simulink model "Sliding_mode_observer"  (R2024b)
settings: Solver=VariableStepAuto  StartTime=0.0  StopTime=10  FixedStep=1e-5  RelTol=1e-3  EnableMultiTasking=on
values from neighbouring files (symbols this model uses):
  Ad = Ts / Ld    (= 0.0178571428571)    [init_params.m]
  Aq = Ts / Lq    (= 0.0178571428571)    [init_params.m]
  Bd = 1-(Rs*Ts/Ld)    (= 0.908928571429)    [init_params.m]
  Bq = 1-(Rs*Ts/Lq)    (= 0.908928571429)    [init_params.m]
  Bs = 1E-5    (= 1e-05)    [init_params.m]
  J = 0.0002    [init_params.m]
  k_sat = 1    [init_params.m]
  k_smo = 8    [init_params.m]
  Ki_current = Rs * bw_current    (= 6408.84901332)    [init_params.m]
  Kp_current = Ld * bw_current    (= 3.51858377202)    [init_params.m]
  Ld = 2.8e-3    (= 0.0028)    [init_params.m]
  Lq = 2.8e-3    (= 0.0028)    [init_params.m]
  Pn = 7    [init_params.m]
  psi_f = 0.0078    [init_params.m]
  Rs = 5.1    [init_params.m]
  Ts = 50e-6    (= 5e-05)    [init_params.m]
undefined symbols (not defined in the file or in its folder): DiscIntNeverNeededParam
libraries: slpidlib x4, eeGeneralControl x4, spsPWMGenerator2LevelLib x1, spsDCVoltageSourceLib x1, spsGroundLib x1, spsPermanentMagnetSynchronousMachineLib x1, spsThreePhaseVIMeasurementLib x1, spsTwoLevelConverterLib x1, spspowerguiLib x1
settings Model: Creator=yangchaojie  LastModifiedBy=yangchaojie
settings SolverCC: PositivePriorityOrder=on  AutoInsertRateTranBlk=on
settings OptimizationCC: DefaultParameterBehavior=Inlined  UseDivisionForNetSlopeComputation=on  GainParamInheritBuiltInType=on  UseFloatMulNetSlope=on  InlineInvariantSignals=on  PassReuseOutputArgsAs=Individual arguments  ZeroExternalMemoryAtStartup=off  ZeroInternalMemoryAtStartup=off  NoFixptDivByZeroProtection=on  EfficientFloat2IntCast=on  LifeSpan=1  MaxStackSize=512  OptimizeBlockOrder=speed  DifferentSizesBufferReuse=on  EfficientTunableParamExpr=on
settings DebuggingCC: ParameterTunabilityLossMsg=error
settings HardwareCC: ProdBitPerPointer=32  ProdBitPerSizeT=32  ProdBitPerPtrDiffT=32  ProdLargestAtomicInteger=Long  ProdLargestAtomicFloat=Double  ProdWordSize=32  ProdLongLongMode=on  ProdHWDeviceType=ARM Compatible->ARM Cortex-M
settings SFSimCC: MATLABDynamicMemAlloc=off
settings RTWCC: Description=Embedded Coder  SystemTargetFile=ert.tlc  GenCodeOnly=on  TemplateMakefile=ert_default_tmf  GenerateReport=on  Toolchain=GNU Tools for ARM Embedded Processors  LaunchReport=on
settings CodeAppCC: ForceParamTrailComments=on  IgnoreCustomStorageClasses=off  OperatorAnnotations=on  SimulinkDataObjDesc=on  SFDataObjDesc=on  CustomSymbolStrGlobalVar=rt$N$M  CustomSymbolStrType=$N$M  CustomSymbolStrFcn=$N$M$F  CustomSymbolStrMacro=$N$M  InsertBlockDesc=on
settings ERTTargetCC: TargetLangStandard=C99 (ISO)  CodeReplacementLibrary=ARM Cortex-M  IncludeMdlTerminateFcn=off  CombineSignalStateStructs=on  SupportAbsoluteTime=off  SupportComplex=off  SupportNonInlinedSFcns=on  ExtModeTransport=3  ExtModeStaticAlloc=on  ExtModeStaticAllocSize=2048  ExtModeMexFile=ext_xcp  ExtModeIntrfLevel=Level2 - Open  ERTCustomFileTemplate=example_file_process.tlc  ERTFilePackagingFormat=CompactWithDataFile

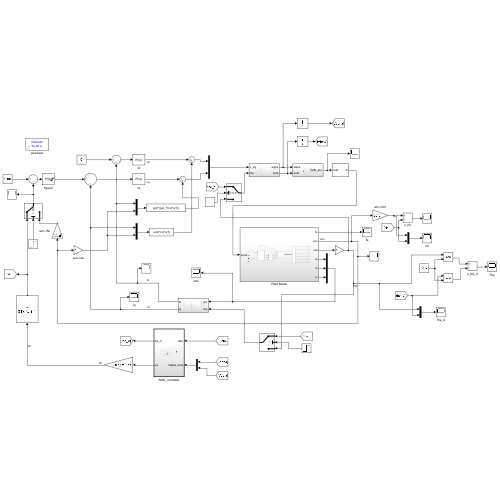
[thumbnail: Simulink's stored preview of the top-level diagram]
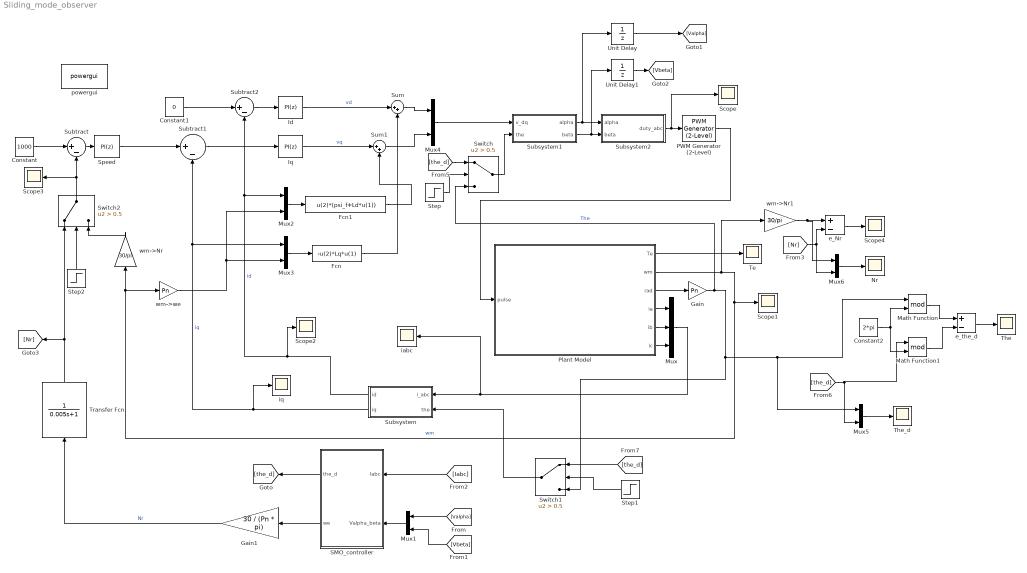
== system Sliding_mode_observer ==
  Constant : Constant  Value=1000
  Constant1 : Constant  Value=0
  Constant2 : Constant  Value=2*pi
  Fcn : Fcn  Expr=-u(2)*Lq*u(1)
  Fcn1 : Fcn  Expr=u(2)*(psi_f+Ld*u(1))
  Gain : Gain  Gain=Pn
  Gain1 : Gain  Gain=30 / (Pn * pi)
  Id : slpidlib/PID Controller  Controller=PI  Form=Parallel  TimeDomain=Discrete-time  UseExternalTs=off  SampleTime=1/10000  IntegratorMethod=Forward Euler  FilterMethod=Forward Euler  ControllerParametersSource=internal  P=Kp_current  I=Ki_current  UseKiTs=off  D=0  UseExternalDerivativeSource=off  N=100  UseFilter=on  TunerSelectOption=Transfer Function Based (PID Tuner App)  InitialConditionSource=internal  InitialConditionForIntegrator=0  InitialConditionForFilter=0  DifferentiatorICPrevScaledInput=0  ExternalReset=none  TrackingMode=off  Kt=1  LimitOutput=off  SatLimitsSource=internal  UpperSaturationLimit=inf  LowerSaturationLimit=-inf  LinearizeAsGain=on  AntiWindupMode=none  Kb=1  LimitIntegrator=off  UpperIntegratorSaturationLimit=inf  LowerIntegratorSaturationLimit=-inf  POutMin=[]  POutMax=[]  IOutMin=[]  IOutMax=[]  DOutMin=[]  DOutMax=[]  NOutMin=[]  NOutMax=[]  SumOutMin=[]  SumOutMax=[]  SaturationOutMin=[]  SaturationOutMax=[]  PParamMin=[]  PParamMax=[]  IParamMin=[]  IParamMax=[]  DParamMin=[]  DParamMax=[]  NParamMin=[]  NParamMax=[]  KbParamMin=[]  KbParamMax=[]  KtParamMin=[]  KtParamMax=[]  KbOutMin=[]  KbOutMax=[]  KtOutMin=[]  KtOutMax=[]  IntegratorOutMin=[]  IntegratorOutMax=[]  FilterOutMin=[]  FilterOutMax=[]  SumI1OutMin=[]  SumI1OutMax=[]  SumI2OutMin=[]  SumI2OutMax=[]  SumI3OutMin=[]  SumI3OutMax=[]  SumI4OutMin=[]  SumI4OutMax=[]  SumDOutMin=[]  SumDOutMax=[]  DifferentiatorOutMin=[]  DifferentiatorOutMax=[]  FilterDiffOutCoefMin=[]  FilterDiffOutCoefMax=[]  ReciprocalOutMin=[]  ReciprocalOutMax=[]  SumDenOutMin=[]  SumDenOutMax=[]  SumNumOutMin=[]  SumNumOutMax=[]  DivideOutMin=[]  DivideOutMax=[]  UdiffTsProdOutMin=[]  UdiffTsProdOutMax=[]  NTsProdOutMin=[]  NTsProdOutMax=[]  UintegralTsProdOutMin=[]  UintegralTsProdOutMax=[]  UngainTsProdOutMin=[]  UngainTsProdOutMax=[]  ClampingZeroOutDataTypeStr=Inherit: Inherit via back propagation  ClampingZeroOutMin=[]  ClampingZeroOutMax=[]  FilterDenConstantOutDataTypeStr=Inherit: Inherit via back propagation  FilterDenConstantOutMin=[]  FilterDenConstantOutMax=[]  PCopyOutDataTypeStr=Inherit: Inherit via back propagation  PCopyOutMin=[]  PCopyOutMax=[]  NCopyOutDataTypeStr=Inherit: Inherit via back propagation  NCopyOutMin=[]  NCopyOutMax=[]  IntegratorContinuousStateAttributes=''  IntegratorStateMustResolveToSignalObject=off  IntegratorRTWStateStorageClass=Auto  FilterContinuousStateAttributes=''  FilterStateMustResolveToSignalObject=off  FilterRTWStateStorageClass=Auto  ParallelPVariant=InternalParameters  IdealPVariant=Disabled  IVariant=InternalParameters  DVariant=Disabled  IntegratorVariant=Discrete  SatVariant=Disabled  AWVariant=Passthrough  PCopyVariant=Disabled  TRVariant=Disabled  FdbkBlocksVariant=Forward  IdealPFdbkVariant=Disabled  SatFdbkVariant=Disabled  DerivativeFilterVariant=Disabled  NVariant=Disabled  NCopyVariant=Disabled_SignalSpec  FilterICVariant=Disabled  IntegratorICVariant=InternalICs  ExternalResetVariant=Disabled  TRSumVariant=Passthrough  SumFdbkVariant=Disabled  SumVariant=Sum_PI  TsampFilterVariant=InternalTs  TsampNgainVariant=Passthrough  TsampIntegralVariant=Disabled_SignalSpec  ExternalSaturationOutDataTypeStr=Inherit: Same as second input  DerivativeSourceVariant=Disabled  PreIntVariant=InternalPreInt
  Iq : slpidlib/PID Controller  Controller=PI  Form=Parallel  TimeDomain=Discrete-time  UseExternalTs=off  SampleTime=1/10000  IntegratorMethod=Forward Euler  FilterMethod=Forward Euler  ControllerParametersSource=internal  P=Kp_current  I=Ki_current  UseKiTs=off  D=0  UseExternalDerivativeSource=off  N=100  UseFilter=on  TunerSelectOption=Transfer Function Based (PID Tuner App)  InitialConditionSource=internal  InitialConditionForIntegrator=0  InitialConditionForFilter=0  DifferentiatorICPrevScaledInput=0  ExternalReset=none  TrackingMode=off  Kt=1  LimitOutput=off  SatLimitsSource=internal  UpperSaturationLimit=inf  LowerSaturationLimit=-inf  LinearizeAsGain=on  AntiWindupMode=none  Kb=1  LimitIntegrator=off  UpperIntegratorSaturationLimit=inf  LowerIntegratorSaturationLimit=-inf  POutMin=[]  POutMax=[]  IOutMin=[]  IOutMax=[]  DOutMin=[]  DOutMax=[]  NOutMin=[]  NOutMax=[]  SumOutMin=[]  SumOutMax=[]  SaturationOutMin=[]  SaturationOutMax=[]  PParamMin=[]  PParamMax=[]  IParamMin=[]  IParamMax=[]  DParamMin=[]  DParamMax=[]  NParamMin=[]  NParamMax=[]  KbParamMin=[]  KbParamMax=[]  KtParamMin=[]  KtParamMax=[]  KbOutMin=[]  KbOutMax=[]  KtOutMin=[]  KtOutMax=[]  IntegratorOutMin=[]  IntegratorOutMax=[]  FilterOutMin=[]  FilterOutMax=[]  SumI1OutMin=[]  SumI1OutMax=[]  SumI2OutMin=[]  SumI2OutMax=[]  SumI3OutMin=[]  SumI3OutMax=[]  SumI4OutMin=[]  SumI4OutMax=[]  SumDOutMin=[]  SumDOutMax=[]  DifferentiatorOutMin=[]  DifferentiatorOutMax=[]  FilterDiffOutCoefMin=[]  FilterDiffOutCoefMax=[]  ReciprocalOutMin=[]  ReciprocalOutMax=[]  SumDenOutMin=[]  SumDenOutMax=[]  SumNumOutMin=[]  SumNumOutMax=[]  DivideOutMin=[]  DivideOutMax=[]  UdiffTsProdOutMin=[]  UdiffTsProdOutMax=[]  NTsProdOutMin=[]  NTsProdOutMax=[]  UintegralTsProdOutMin=[]  UintegralTsProdOutMax=[]  UngainTsProdOutMin=[]  UngainTsProdOutMax=[]  ClampingZeroOutDataTypeStr=Inherit: Inherit via back propagation  ClampingZeroOutMin=[]  ClampingZeroOutMax=[]  FilterDenConstantOutDataTypeStr=Inherit: Inherit via back propagation  FilterDenConstantOutMin=[]  FilterDenConstantOutMax=[]  PCopyOutDataTypeStr=Inherit: Inherit via back propagation  PCopyOutMin=[]  PCopyOutMax=[]  NCopyOutDataTypeStr=Inherit: Inherit via back propagation  NCopyOutMin=[]  NCopyOutMax=[]  IntegratorContinuousStateAttributes=''  IntegratorStateMustResolveToSignalObject=off  IntegratorRTWStateStorageClass=Auto  FilterContinuousStateAttributes=''  FilterStateMustResolveToSignalObject=off  FilterRTWStateStorageClass=Auto  ParallelPVariant=InternalParameters  IdealPVariant=Disabled  IVariant=InternalParameters  DVariant=Disabled  IntegratorVariant=Discrete  SatVariant=Disabled  AWVariant=Passthrough  PCopyVariant=Disabled  TRVariant=Disabled  FdbkBlocksVariant=Forward  IdealPFdbkVariant=Disabled  SatFdbkVariant=Disabled  DerivativeFilterVariant=Disabled  NVariant=Disabled  NCopyVariant=Disabled_SignalSpec  FilterICVariant=Disabled  IntegratorICVariant=InternalICs  ExternalResetVariant=Disabled  TRSumVariant=Passthrough  SumFdbkVariant=Disabled  SumVariant=Sum_PI  TsampFilterVariant=InternalTs  TsampNgainVariant=Passthrough  TsampIntegralVariant=Disabled_SignalSpec  ExternalSaturationOutDataTypeStr=Inherit: Same as second input  DerivativeSourceVariant=Disabled  PreIntVariant=InternalPreInt
  Math Function : Math  Operator=mod
  Math Function1 : Math  Operator=mod
  Mux : Mux  Inputs=3
  Mux{1..6} (6 alike) : Mux  Inputs=2
  Nr : Scope
  PWM Generator (2-Level) : spsPWMGenerator2LevelLib/PWM Generator (2-Level)  ModulatorType=Three-phase bridge (6 pulses)  ModulatorMode=Unsynchronized  Fc=10000  Pc=90  nF=27  MinMax="[ -1  1 ]"  SamplingTechnique=Natural  ModulatingSignals=off  m=0.8  Freq=60  Phase=0  Ts=0  ShowCarrierOutport=off
  Plant Model : Subsystem
  SMO_controller : Subsystem  TreatAsAtomicUnit=on
  Scope{,1..4} (5 alike) : Scope
  Speed : slpidlib/PID Controller  Controller=PI  Form=Parallel  TimeDomain=Discrete-time  UseExternalTs=off  SampleTime=1/1000  IntegratorMethod=Forward Euler  FilterMethod=Forward Euler  ControllerParametersSource=internal  P=0.05  I=0.005  UseKiTs=off  D=0  UseExternalDerivativeSource=off  N=100  UseFilter=on  TunerSelectOption=Transfer Function Based (PID Tuner App)  InitialConditionSource=internal  InitialConditionForIntegrator=0  InitialConditionForFilter=0  DifferentiatorICPrevScaledInput=0  ExternalReset=none  TrackingMode=off  Kt=1  LimitOutput=on  SatLimitsSource=internal  UpperSaturationLimit=2  LowerSaturationLimit=-2  LinearizeAsGain=on  AntiWindupMode=none  Kb=1  LimitIntegrator=off  UpperIntegratorSaturationLimit=inf  LowerIntegratorSaturationLimit=-inf  POutMin=[]  POutMax=[]  IOutMin=[]  IOutMax=[]  DOutMin=[]  DOutMax=[]  NOutMin=[]  NOutMax=[]  SumOutMin=[]  SumOutMax=[]  SaturationOutMin=[]  SaturationOutMax=[]  PParamMin=[]  PParamMax=[]  IParamMin=[]  IParamMax=[]  DParamMin=[]  DParamMax=[]  NParamMin=[]  NParamMax=[]  KbParamMin=[]  KbParamMax=[]  KtParamMin=[]  KtParamMax=[]  KbOutMin=[]  KbOutMax=[]  KtOutMin=[]  KtOutMax=[]  IntegratorOutMin=[]  IntegratorOutMax=[]  FilterOutMin=[]  FilterOutMax=[]  SumI1OutMin=[]  SumI1OutMax=[]  SumI2OutMin=[]  SumI2OutMax=[]  SumI3OutMin=[]  SumI3OutMax=[]  SumI4OutMin=[]  SumI4OutMax=[]  SumDOutMin=[]  SumDOutMax=[]  DifferentiatorOutMin=[]  DifferentiatorOutMax=[]  FilterDiffOutCoefMin=[]  FilterDiffOutCoefMax=[]  ReciprocalOutMin=[]  ReciprocalOutMax=[]  SumDenOutMin=[]  SumDenOutMax=[]  SumNumOutMin=[]  SumNumOutMax=[]  DivideOutMin=[]  DivideOutMax=[]  UdiffTsProdOutMin=[]  UdiffTsProdOutMax=[]  NTsProdOutMin=[]  NTsProdOutMax=[]  UintegralTsProdOutMin=[]  UintegralTsProdOutMax=[]  UngainTsProdOutMin=[]  UngainTsProdOutMax=[]  ClampingZeroOutDataTypeStr=Inherit: Inherit via back propagation  ClampingZeroOutMin=[]  ClampingZeroOutMax=[]  FilterDenConstantOutDataTypeStr=Inherit: Inherit via back propagation  FilterDenConstantOutMin=[]  FilterDenConstantOutMax=[]  PCopyOutDataTypeStr=Inherit: Inherit via back propagation  PCopyOutMin=[]  PCopyOutMax=[]  NCopyOutDataTypeStr=Inherit: Inherit via back propagation  NCopyOutMin=[]  NCopyOutMax=[]  IntegratorContinuousStateAttributes=''  IntegratorStateMustResolveToSignalObject=off  IntegratorRTWStateStorageClass=Auto  FilterContinuousStateAttributes=''  FilterStateMustResolveToSignalObject=off  FilterRTWStateStorageClass=Auto  ParallelPVariant=InternalParameters  IdealPVariant=Disabled  IVariant=InternalParameters  DVariant=Disabled  IntegratorVariant=Discrete  SatVariant=Enabled  AWVariant=Passthrough  PCopyVariant=Disabled  TRVariant=Disabled  FdbkBlocksVariant=Forward  IdealPFdbkVariant=Disabled  SatFdbkVariant=Disabled  DerivativeFilterVariant=Disabled  NVariant=Disabled  NCopyVariant=Disabled_SignalSpec  FilterICVariant=Disabled  IntegratorICVariant=InternalICs  ExternalResetVariant=Disabled  TRSumVariant=Passthrough  SumFdbkVariant=Disabled  SumVariant=Sum_PI  TsampFilterVariant=InternalTs  TsampNgainVariant=Passthrough  TsampIntegralVariant=Disabled_SignalSpec  ExternalSaturationOutDataTypeStr=Inherit: Same as second input  DerivativeSourceVariant=Disabled  PreIntVariant=InternalPreInt
  Step : Step  Time=5  SampleTime=0
  Step1 : Step  Time=5  SampleTime=0
  Step2 : Step  Time=5  SampleTime=0
  Subsystem : Subsystem
  Subsystem1 : Subsystem
  Subsystem2 : Subsystem
  Subtract : Sum  Inputs=|+-
  Subtract1 : Sum  Inputs=|+-
  Subtract2 : Sum  Inputs=|+-
  Sum : Sum  Inputs=|++
  Sum1 : Sum  Inputs=|++
  Switch : Switch  Criteria=u2 > Threshold  Threshold=0.5  SaturateOnIntegerOverflow=off  InputSameDT=off
  Switch1 : Switch  Criteria=u2 > Threshold  Threshold=0.5  SaturateOnIntegerOverflow=off  InputSameDT=off
  Switch2 : Switch  Criteria=u2 > Threshold  Threshold=0.5  SaturateOnIntegerOverflow=off  InputSameDT=off
  Te : Scope
  The : Scope
  The_d : Scope
  Transfer Fcn : TransferFcn  Denominator="[0.005  1]"
  Unit Delay : UnitDelay  SampleTime=Ts  HasFrameUpgradeWarning=on
  Unit Delay1 : UnitDelay  SampleTime=Ts  HasFrameUpgradeWarning=on
  e_Nr : Sum  Inputs=+-
  e_the_d : Sum  Inputs=+-
  iabc : Scope
  iq : Scope
  powergui : spspowerguiLib/powergui  Priority=1  SimulationMode=Discrete  SampleTime=Ts  frequency=60  Iterations=50  frequencyindice=0  Pbase=100e6  ErrMax=1e-4  UnitsV=kV  UnitsW=MW  buscounter=0  FunctionMessages=off  echomessages=off  EnableUseOfTLC=off  CurrentSourceSwitches=off  DisableSnubberDevices=off  DisableRonSwitches=off  DisableVfSwitches=off  DisplayEquations=off  AutomaticDiscreteSolvers=off  SolverType=Tustin/Backward Euler (TBE)  Interpol=off  ExternalGateDelay=off  methode=off  Ts=100  x0status=blocks  SPID=on  SwTol=0  HookPort=off  NonlinearTolerance=1e-4  nMaxIteration=100  ContinueOnMaxIteration=off  RestoreLinks=warning  ResistiveCurrentMeasurement=off  Frange=[0:2:500]  Ylog=off  Xlog=on  ShowGrid=off  save=off  variable=ZData  structure=0  ZoomFFT=off  StartTime=0.0  cycles=1  DisplayStyle=1  fundamental=60  FreqAxis=off  MaxFrequency=1000  frequencyindicesteady=1  RmsSteady=1  display=off
  wm->Nr : Gain  Gain=30/pi
  wm->Nr1 : Gain  Gain=30/pi
  wm->we : Gain  Gain=Pn
  wires:
  SMO_controller/2(we) -> Gain1/1
  SMO_controller/1(the_d) -> [the_d]
  Gain1/1 -> Transfer Fcn/1  "Nr"
  Plant Model/6(ic) -> Mux/3
  Plant Model/5(ib) -> Mux/2
  Fcn1/1 -> Sum1/2
  Plant Model/2(wm) -> wm->Nr1/1, Scope1/1, wm->Nr/1, wm->we/1  "wm"
  Constant/1 -> Subtract/1
  Subtract1/1 -> Iq/1
  Iq/1 -> Sum1/1  "vq"
  Subsystem/1(id) -> Mux2/1, Subtract2/2, Scope2/1  "id"
  Mux/1 -> iabc/1, Subsystem/1(i_abc)
  Constant1/1 -> Subtract2/1
  Mux4/1 -> Subsystem1/1(v_dq)
  Subsystem1/2(beta) -> Unit Delay1/1, Subsystem2/2(beta)
  Sum1/1 -> Mux4/2
  Subtract2/1 -> Id/1
  PWM Generator (2-Level)/1 -> Plant Model/1(pulse)
  Mux2/1 -> Fcn1/1
  Plant Model/1(Te) -> Te/1
  wm->we/1 -> Mux3/2, Mux2/2
  Plant Model/4(ia) -> Mux/1
  Subsystem/2(iq) -> iq/1, Mux3/1, Subtract1/2  "iq"
  Fcn/1 -> Sum/2
  Sum/1 -> Mux4/1
  Gain/1 -> Switch/3, Switch1/3, Math Function/1, Mux5/1  "The"
  Plant Model/3(rad) -> Gain/1
  Mux3/1 -> Fcn/1
  Subtract/1 -> Speed/1
  Subsystem1/1(alpha) -> Unit Delay/1, Subsystem2/1(alpha)
  Id/1 -> Sum/1  "vd"
  Speed/1 -> Subtract1/1
  Subsystem2/1(duty_abc) -> PWM Generator (2-Level)/1, Scope/1
  Mux1/1 -> SMO_controller/2(Valpha_beta)
  [Valpha] -> Mux1/1
  [Vbeta] -> Mux1/2
  [Iabc] -> SMO_controller/1(Iabc)
  e_Nr/1 -> Scope4/1
  wm->Nr1/1 -> Mux6/1, e_Nr/1
  [Nr] -> Mux6/2, e_Nr/2
  Unit Delay/1 -> [Valpha]
  Unit Delay1/1 -> [Vbeta]
  [the_d] -> Switch/1
  Switch/1 -> Subsystem1/2(the)
  Switch1/1 -> Subsystem/2(the)
  Switch2/1 -> Subtract/2, Scope3/1
  wm->Nr/1 -> Switch2/3
  [the_d] -> Math Function1/1, Mux5/2
  e_the_d/1 -> The/1
  Step/1 -> Switch/2
  [the_d] -> Switch1/1
  Step1/1 -> Switch1/2
  Step2/1 -> Switch2/2
  Mux5/1 -> The_d/1
  Mux6/1 -> Nr/1
  Transfer Fcn/1 -> Switch2/1, [Nr]
  Constant2/1 -> Math Function/2, Math Function1/2
  Math Function/1 -> e_the_d/1
  Math Function1/1 -> e_the_d/2

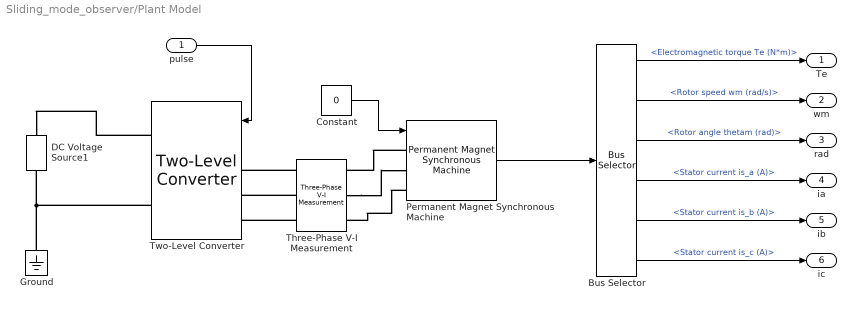
== system Sliding_mode_observer/Plant Model ==
  pulse : Inport
  Bus Selector : BusSelector  OutputSignals=Electromagnetic torque Te (N*m),Rotor speed wm (rad/s),Rotor angle thetam (rad),Stator current is_a (A),Stator current is_b (A),Stator current is_c (A)
  Constant : Constant  Value=0
  DC Voltage Source1 : spsDCVoltageSourceLib/DC Voltage Source  Amplitude=12  Measurements=None
  Ground : spsGroundLib/Ground  LConnTagsString=a
  Permanent Magnet Synchronous Machine : spsPermanentMagnetSynchronousMachineLib/Permanent Magnet Synchronous Machine  NbPhases=3  FluxDistribution=Sinusoidal  RotorType=Round  MechanicalLoad=Torque Tm  PresetModel=No  ShowDetailedParameters=on  MeasurementBus=off  Resistance=Rs  Inductance=8.5e-3  dqInductances=[8.5e-3,8.5e-3]  La=Ld  MachineConstant=Flux linkage established by magnets (V.s)  Flux=psi_f  VoltageCst=9.9033  TorqueCst=0.0819  Flat=120  Mechanical=[J Bs Pn 0]  PolePairs=4  InitialConditions=[0,0, 0,0]  InitialConditions5ph=[0 0 0 0 0 0]  RefAngle=Aligned with phase A axis (original Park)  IterativeDiscreteModel=Trapezoidal non iterative  TsBlock=-1  TsPowergui=0
  Three-Phase V-I Measurement : spsThreePhaseVIMeasurementLib/Three-Phase V-I Measurement  VoltageMeasurement=phase-to-ground  SetLabelV=on  LabelV=Vabc  Vpu=off  VpuLL=off  CurrentMeasurement=yes  SetLabelI=on  LabelI=Iabc  Ipu=off  Pbase=100e6  Vbase=500e3  OutputType=Complex  PhasorSimulation=off  PSBequivalent=0
  Two-Level Converter : spsTwoLevelConverterLib/Two-Level Converter  ModelType=Switching devices  Ron=1e-3  Rs=1e6  Cs=inf  Vforward=[0,0]  Ron_Diode=1e-3  Rs_Diode=1e6  Cs_Diode=inf  Vf_Diode=1e-3  Rs_CurrentSource=inf  Ron_ACsource=1e-3
  Te : Outport
  wm : Outport  Port=2
  rad : Outport  Port=3
  ia : Outport  Port=4
  ib : Outport  Port=5
  ic : Outport  Port=6
  wires:
  pulse/1 -> Two-Level Converter/1
  Permanent Magnet Synchronous Machine/1 -> Bus Selector/1
  Bus Selector/1 -> Te/1  "<Electromagnetic torque Te (N*m)>"
  Bus Selector/2 -> wm/1  "<Rotor speed wm (rad/s)>"
  Bus Selector/6 -> ic/1  "<Stator current is_c (A)>"
  Bus Selector/5 -> ib/1  "<Stator current is_b (A)>"
  Bus Selector/4 -> ia/1  "<Stator current is_a (A)>"
  Bus Selector/3 -> rad/1  "<Rotor angle thetam (rad)>"
  Constant/1 -> Permanent Magnet Synchronous Machine/1
  connections:
  Two-Level Converter/RConn1 -- DC Voltage Source1/RConn1
  Two-Level Converter/RConn2 -- Ground/LConn1 -- DC Voltage Source1/LConn1
  Permanent Magnet Synchronous Machine/LConn1 -- Three-Phase V-I Measurement/RConn1
  Three-Phase V-I Measurement/LConn1 -- Two-Level Converter/LConn1
  Three-Phase V-I Measurement/LConn2 -- Two-Level Converter/LConn2
  Three-Phase V-I Measurement/LConn3 -- Two-Level Converter/LConn3
  Three-Phase V-I Measurement/RConn2 -- Permanent Magnet Synchronous Machine/LConn2
  Permanent Magnet Synchronous Machine/LConn3 -- Three-Phase V-I Measurement/RConn3

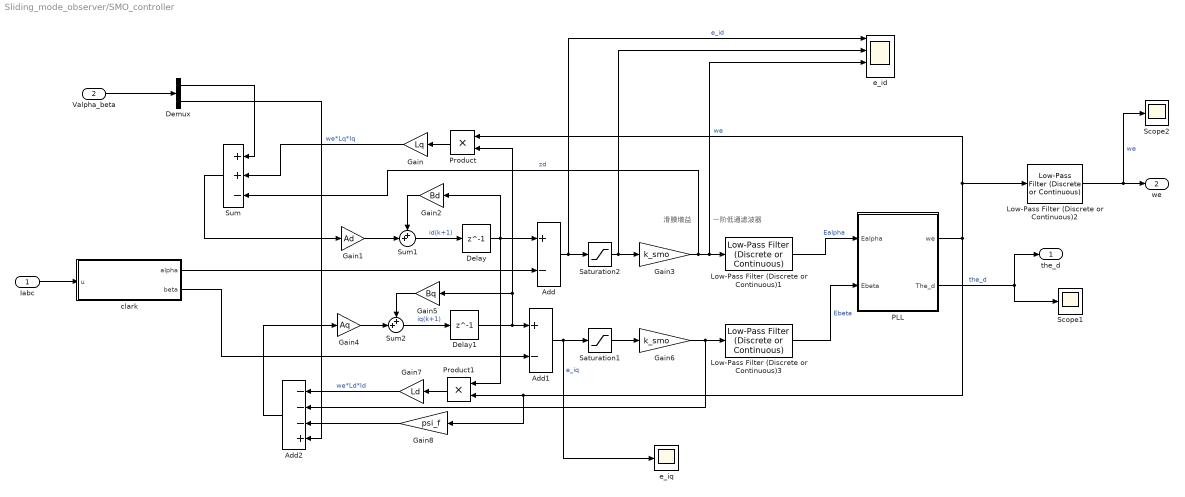
== system Sliding_mode_observer/SMO_controller ==
  note: 一阶低通滤波器
  note: 滑膜增益
  Iabc : Inport
  Valpha_beta : Inport  Port=2
  Add : Sum  Inputs=+-
  Add1 : Sum  Inputs=+-
  Add2 : Sum  Inputs=---+
  Delay : Delay  DelayLength=1  InputProcessing=Columns as channels (frame based)  SampleTime=Ts
  Delay1 : Delay  DelayLength=1  InputProcessing=Columns as channels (frame based)  SampleTime=Ts
  Demux : Demux  Outputs=2
  Gain : Gain  Gain=Lq
  Gain1 : Gain  Gain=Ad
  Gain2 : Gain  Gain=Bd
  Gain3 : Gain  Gain=k_smo
  Gain4 : Gain  Gain=Aq
  Gain5 : Gain  Gain=Bq
  Gain6 : Gain  Gain=k_smo
  Gain7 : Gain  Gain=Ld
  Gain8 : Gain  Gain=psi_f
  Low-Pass Filter (Discrete or Continuous)1 : eeGeneralControl/Low-Pass Filter (Discrete or Continuous)  K=1  T=0.0005  B=inf  A=-inf  init_option=Inherited from block input  x0=0  Ts=Ts
  Low-Pass Filter (Discrete or Continuous)2 : eeGeneralControl/Low-Pass Filter (Discrete or Continuous)  K=1  T=0.0008  B=inf  A=-inf  init_option=Inherited from block input  x0=0  Ts=Ts
  Low-Pass Filter (Discrete or Continuous)3 : eeGeneralControl/Low-Pass Filter (Discrete or Continuous)  K=1  T=0.0005  B=inf  A=-inf  init_option=Inherited from block input  x0=0  Ts=Ts
  PLL : Subsystem
  Product : Product
  Product1 : Product
  Saturation1 : Saturate  UpperLimit=k_sat  LowerLimit=-k_sat
  Saturation2 : Saturate  UpperLimit=k_sat  LowerLimit=-k_sat
  Scope1 : Scope
  Scope2 : Scope
  Sum : Sum  Inputs=++-
  Sum1 : Sum  Inputs=++|
  Sum2 : Sum  Inputs=++|
  clark : MATLAB Function  TreatAsAtomicUnit=on
  e_id : Scope  NumInputPorts=4
  e_iq : Scope
  the_d : Outport
  we : Outport  Port=2
  wires:
  Delay1/1 -> Product/2, Gain5/1, Add1/1
  Gain4/1 -> Sum2/2
  Add2/1 -> Gain4/1
  Add/1 -> Saturation2/1, e_id/1  "e_id"
  Gain7/1 -> Add2/1  "we*Ld*Id"
  Product/1 -> Gain/1
  Product1/1 -> Gain7/1
  Sum2/1 -> Delay1/1  "iq(k+1)"
  Gain/1 -> Sum/2  "we*Lq*Iq"
  Delay/1 -> Product1/1, Add/1, Gain2/1
  Sum/1 -> Gain1/1
  Sum1/1 -> Delay/1  "id(k+1)"
  Gain2/1 -> Sum1/1
  Gain1/1 -> Sum1/2
  Gain5/1 -> Sum2/1
  Gain3/1 -> Sum/3, e_id/3, Low-Pass Filter (Discrete or Continuous)1/1  "zd"
  Add1/1 -> Saturation1/1, e_iq/1  "e_iq"
  Valpha_beta/1 -> Demux/1
  PLL/2(The_d) -> the_d/1, Scope1/1  "the_d"
  Gain8/1 -> Add2/3
  Low-Pass Filter (Discrete or Continuous)2/1 -> Scope2/1, we/1  "we"
  PLL/1(we) -> Product/1, Low-Pass Filter (Discrete or Continuous)2/1, Gain8/1, Product1/2  "we"
  Gain6/1 -> Add2/2, Low-Pass Filter (Discrete or Continuous)3/1
  clark/2(beta) -> Add1/2
  Saturation2/1 -> Gain3/1, e_id/2
  Saturation1/1 -> Gain6/1
  Demux/1 -> Sum/1
  Demux/2 -> Add2/4
  Iabc/1 -> clark/1(u)
  clark/1(alpha) -> Add/2
  Low-Pass Filter (Discrete or Continuous)1/1 -> PLL/1(Ealpha)  "Ealpha"
  Low-Pass Filter (Discrete or Continuous)3/1 -> PLL/2(Ebeta)  "Ebeta"

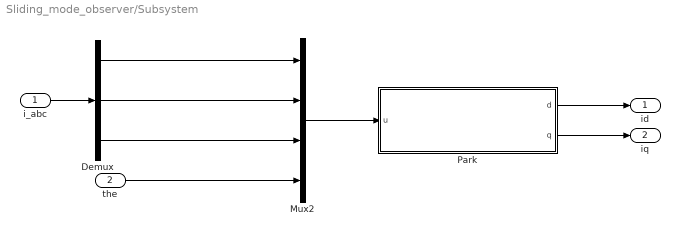
== system Sliding_mode_observer/Subsystem ==
  i_abc : Inport
  the : Inport  Port=2
  Demux : Demux  Outputs=3
  Mux2 : Mux
  Park : MATLAB Function  TreatAsAtomicUnit=on
  id : Outport
  iq : Outport  Port=2
  wires:
  Mux2/1 -> Park/1(u)
  Park/2(q) -> iq/1
  the/1 -> Mux2/4
  Park/1(d) -> id/1
  Demux/1 -> Mux2/1
  Demux/2 -> Mux2/2
  Demux/3 -> Mux2/3
  i_abc/1 -> Demux/1

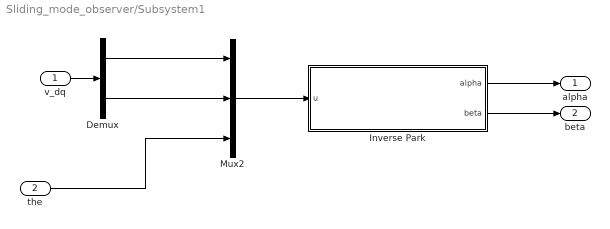
== system Sliding_mode_observer/Subsystem1 ==
  v_dq : Inport
  the : Inport  Port=2
  Demux : Demux  Outputs=2
  Inverse Park : MATLAB Function  TreatAsAtomicUnit=on
  Mux2 : Mux  Inputs=3
  alpha : Outport
  beta : Outport  Port=2
  wires:
  Inverse Park/1(alpha) -> alpha/1
  Inverse Park/2(beta) -> beta/1
  Mux2/1 -> Inverse Park/1(u)
  the/1 -> Mux2/3
  Demux/1 -> Mux2/1
  Demux/2 -> Mux2/2
  v_dq/1 -> Demux/1

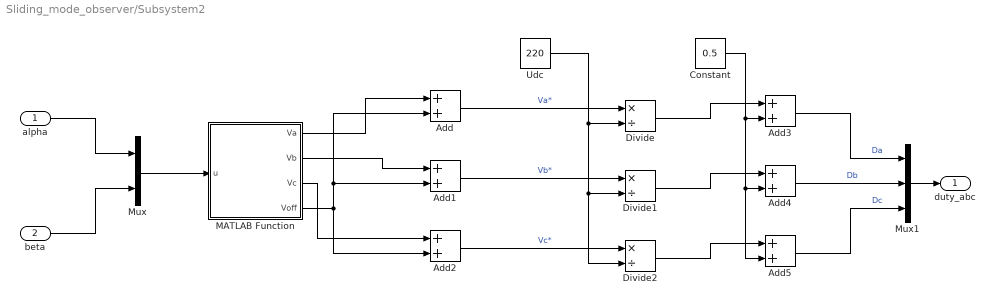
== system Sliding_mode_observer/Subsystem2 ==
  alpha : Inport
  beta : Inport  Port=2
  Add{,1..5} (6 alike) : Sum
  Constant : Constant  Value=0.5
  Divide : Product  Inputs=*/
  Divide1 : Product  Inputs=*/
  Divide2 : Product  Inputs=*/
  MATLAB Function : MATLAB Function  TreatAsAtomicUnit=on
  Mux : Mux  Inputs=2
  Mux1 : Mux  Inputs=3
  Udc : Constant  Value=220
  duty_abc : Outport
  wires:
  Add1/1 -> Divide1/1  "Vb*"
  Udc/1 -> Divide2/2, Divide1/2, Divide/2
  Constant/1 -> Add5/2, Add4/2, Add3/2
  Add3/1 -> Mux1/1  "Da"
  MATLAB Function/4(Voff) -> Add2/2, Add1/2, Add/2
  Add5/1 -> Mux1/3  "Dc"
  Divide1/1 -> Add4/1
  MATLAB Function/3(Vc) -> Add2/1
  alpha/1 -> Mux/1
  Add2/1 -> Divide2/1  "Vc*"
  beta/1 -> Mux/2
  Divide/1 -> Add3/1
  Add4/1 -> Mux1/2  "Db"
  Add/1 -> Divide/1  "Va*"
  MATLAB Function/2(Vb) -> Add1/1
  MATLAB Function/1(Va) -> Add/1
  Mux/1 -> MATLAB Function/1(u)
  Divide2/1 -> Add5/1
  Mux1/1 -> duty_abc/1

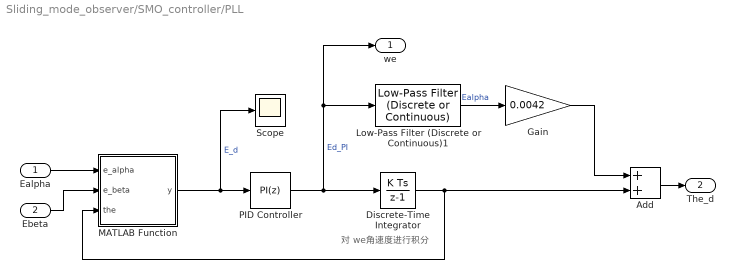
== system Sliding_mode_observer/SMO_controller/PLL ==
  note: 对 we角速度进行积分
  Ealpha : Inport
  Ebeta : Inport  Port=2
  Add : Sum
  Discrete-Time Integrator : DiscreteIntegrator  InitialCondition=-1  SampleTime=Ts  ICPrevOutput=DiscIntNeverNeededParam  ICPrevScaledInput=DiscIntNeverNeededParam
  Gain : Gain  Gain=0.0042
  Low-Pass Filter (Discrete or Continuous)1 : eeGeneralControl/Low-Pass Filter (Discrete or Continuous)  K=1  T=0.0005  B=inf  A=-inf  init_option=Inherited from block input  x0=0  Ts=Ts
  MATLAB Function : MATLAB Function  TreatAsAtomicUnit=on
  PID Controller : slpidlib/PID Controller  Controller=PI  Form=Parallel  TimeDomain=Discrete-time  UseExternalTs=off  SampleTime=Ts  IntegratorMethod=Forward Euler  FilterMethod=Forward Euler  ControllerParametersSource=internal  P=-20  I=-1000  UseKiTs=off  D=0  UseExternalDerivativeSource=off  N=100  UseFilter=on  TunerSelectOption=Transfer Function Based (PID Tuner App)  InitialConditionSource=internal  InitialConditionForIntegrator=0  InitialConditionForFilter=0  DifferentiatorICPrevScaledInput=0  ExternalReset=none  TrackingMode=off  Kt=1  LimitOutput=off  SatLimitsSource=internal  UpperSaturationLimit=4500  LowerSaturationLimit=-4500  LinearizeAsGain=on  AntiWindupMode=clamping  Kb=1  LimitIntegrator=off  UpperIntegratorSaturationLimit=inf  LowerIntegratorSaturationLimit=-inf  POutMin=[]  POutMax=[]  IOutMin=[]  IOutMax=[]  DOutMin=[]  DOutMax=[]  NOutMin=[]  NOutMax=[]  SumOutMin=[]  SumOutMax=[]  SaturationOutMin=[]  SaturationOutMax=[]  PParamMin=[]  PParamMax=[]  IParamMin=[]  IParamMax=[]  DParamMin=[]  DParamMax=[]  NParamMin=[]  NParamMax=[]  KbParamMin=[]  KbParamMax=[]  KtParamMin=[]  KtParamMax=[]  KbOutMin=[]  KbOutMax=[]  KtOutMin=[]  KtOutMax=[]  IntegratorOutMin=[]  IntegratorOutMax=[]  FilterOutMin=[]  FilterOutMax=[]  SumI1OutMin=[]  SumI1OutMax=[]  SumI2OutMin=[]  SumI2OutMax=[]  SumI3OutMin=[]  SumI3OutMax=[]  SumI4OutMin=[]  SumI4OutMax=[]  SumDOutMin=[]  SumDOutMax=[]  DifferentiatorOutMin=[]  DifferentiatorOutMax=[]  FilterDiffOutCoefMin=[]  FilterDiffOutCoefMax=[]  ReciprocalOutMin=[]  ReciprocalOutMax=[]  SumDenOutMin=[]  SumDenOutMax=[]  SumNumOutMin=[]  SumNumOutMax=[]  DivideOutMin=[]  DivideOutMax=[]  UdiffTsProdOutMin=[]  UdiffTsProdOutMax=[]  NTsProdOutMin=[]  NTsProdOutMax=[]  UintegralTsProdOutMin=[]  UintegralTsProdOutMax=[]  UngainTsProdOutMin=[]  UngainTsProdOutMax=[]  ClampingZeroOutDataTypeStr=Inherit: Inherit via back propagation  ClampingZeroOutMin=[]  ClampingZeroOutMax=[]  FilterDenConstantOutDataTypeStr=Inherit: Inherit via back propagation  FilterDenConstantOutMin=[]  FilterDenConstantOutMax=[]  PCopyOutDataTypeStr=Inherit: Inherit via back propagation  PCopyOutMin=[]  PCopyOutMax=[]  NCopyOutDataTypeStr=Inherit: Inherit via back propagation  NCopyOutMin=[]  NCopyOutMax=[]  IntegratorContinuousStateAttributes=''  IntegratorStateMustResolveToSignalObject=off  IntegratorRTWStateStorageClass=Auto  FilterContinuousStateAttributes=''  FilterStateMustResolveToSignalObject=off  FilterRTWStateStorageClass=Auto  ParallelPVariant=InternalParameters  IdealPVariant=Disabled  IVariant=InternalParameters  DVariant=Disabled  IntegratorVariant=Discrete  SatVariant=Disabled  AWVariant=Passthrough  PCopyVariant=Disabled  TRVariant=Disabled  FdbkBlocksVariant=Forward  IdealPFdbkVariant=Disabled  SatFdbkVariant=Disabled  DerivativeFilterVariant=Disabled  NVariant=Disabled  NCopyVariant=Disabled_SignalSpec  FilterICVariant=Disabled  IntegratorICVariant=InternalICs  ExternalResetVariant=Disabled  TRSumVariant=Passthrough  SumFdbkVariant=Disabled  SumVariant=Sum_PI  TsampFilterVariant=InternalTs  TsampNgainVariant=Passthrough  TsampIntegralVariant=Disabled_SignalSpec  ExternalSaturationOutDataTypeStr=Inherit: Same as second input  DerivativeSourceVariant=Disabled  PreIntVariant=InternalPreInt
  Scope : Scope
  we : Outport
  The_d : Outport  Port=2
  wires:
  PID Controller/1 -> we/1, Low-Pass Filter (Discrete or Continuous)1/1, Discrete-Time Integrator/1  "Ed_PI"
  MATLAB Function/1(y) -> Scope/1, PID Controller/1  "E_d"
  Discrete-Time Integrator/1 -> Add/2, MATLAB Function/3(the)
  Ealpha/1 -> MATLAB Function/1(e_alpha)
  Ebeta/1 -> MATLAB Function/2(e_beta)
  Add/1 -> The_d/1
  Low-Pass Filter (Discrete or Continuous)1/1 -> Gain/1  "Ealpha"
  Gain/1 -> Add/1

== matlab function Sliding_mode_observer/Subsystem1/Inverse Park ==
  data: alpha output; beta output; u input
function [alpha, beta] = inverse_park_transform(u)

    alpha = u(1)*cos(u(3))-u(2)*sin(u(3));

    beta = u(1)*sin(u(3))+u(2)*cos(u(3));

end

== matlab function Sliding_mode_observer/Subsystem/Park ==
  data: d output; q output; u input
function [d, q] = park_transform(u)

    d = ((u(1)*cos(u(4))) + u(2)*cos(u(4)-2/3*pi) + u(3)*cos( u(4)+2/3*pi)) * 2/3 ;

    q = -((u(1) * sin(u(4))) + u(2)*sin(u(4)-2/3*pi) + u(3)*sin( u(4) + 2/3*pi )) * 2/3;

end

== matlab function Sliding_mode_observer/Subsystem2/MATLAB Function ==
  data: u input; Va output; Vb output; Vc output; Voff output
function [Va,Vb,Vc,Voff] = fcn(u)

Va = u(1);

Vb = -0.5*u(1)+sqrt(3/4)*u(2);

Vc = -0.5*u(1)-sqrt(3/4)*u(2);

Voff = -0.5*(max([Va,Vb,Vc])+min([Va,Vb,Vc]));

== matlab function Sliding_mode_observer/SMO_controller/PLL/MATLAB Function ==
  data: e_alpha input; y output; e_beta input; the input
function y = park(e_alpha, e_beta, the)

y = e_alpha*cos(the) + e_beta*sin(the);

end

== matlab function Sliding_mode_observer/SMO_controller/clark ==
  data: u input; alpha output; beta output
function [alpha, beta] = clark_transform(u)
    % u 是一个包含三个元素的向量：[u(1), u(2), u(3)]

    % 计算 Alpha
    alpha = (u(1) - 0.5 * (u(2) + u(3))) * (2/3);

    % 计算 Beta
    beta = (sqrt(3)/2 * (u(2) - u(3))) * (2/3);
end
